simulink model "2DoF Robotic Arm"  (R2024b)
settings: Solver=VariableStepAuto  StartTime=0.0  StopTime=10.0  RelTol=1e-3
model workspace: external: MATLAB File C:\Users\sudhi\Downloads\Sagar_Pathak\IIT_Bhilai\Robotics\Assembly_trial_6_DataFile.m (data not in the file)
undefined symbols (not defined in the file): smiData, X, Y, Z
libraries: sm_lib x19, simulink x7, nesl_utility x3
settings Model: PacingRate=1.100000  Creator=sudhi  LastModifiedBy=sudhi

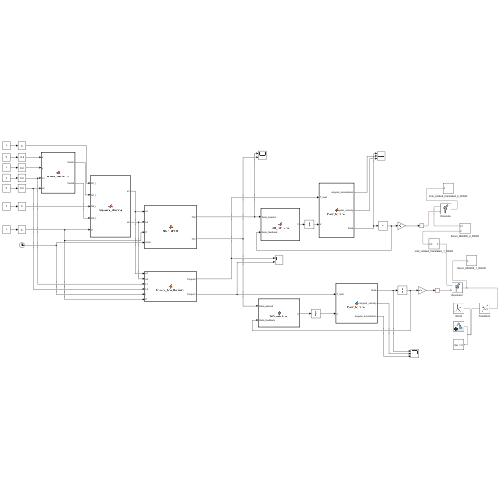
[thumbnail: Simulink's stored preview of the top-level diagram]
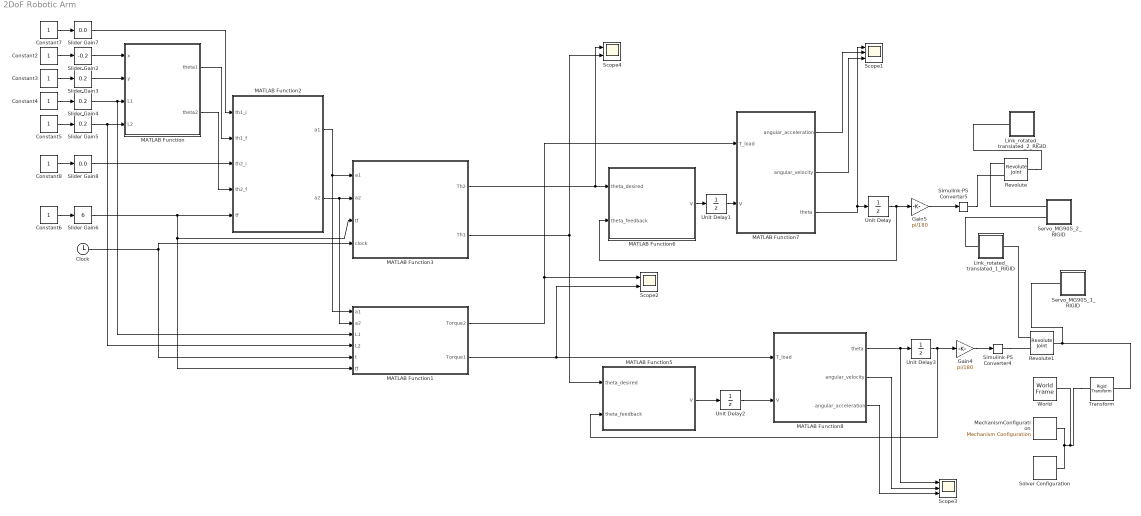
== system 2DoF Robotic Arm ==
  Clock : Clock
  Constant{2..8} (7 alike) : Constant
  Gain4 : Gain  Gain=pi/180
  Gain5 : Gain  Gain=pi/180
  Link_rotated_translated_1_RIGID : Subsystem
  Link_rotated_translated_2_RIGID : Subsystem
  MATLAB Function : MATLAB Function  TreatAsAtomicUnit=on
  MATLAB Function1 : MATLAB Function  TreatAsAtomicUnit=on
  MATLAB Function2 : MATLAB Function  TreatAsAtomicUnit=on
  MATLAB Function3 : MATLAB Function  TreatAsAtomicUnit=on
  MATLAB Function5 : MATLAB Function  TreatAsAtomicUnit=on
  MATLAB Function6 : MATLAB Function  TreatAsAtomicUnit=on
  MATLAB Function7 : MATLAB Function  TreatAsAtomicUnit=on
  MATLAB Function8 : MATLAB Function  TreatAsAtomicUnit=on
  MechanismConfiguration : sm_lib/Utilities/Mechanism Configuration  UniformGravity=Constant  GravityVector=[0 -9.80665 0]  GravityVectorUnits=m/s^2  LinearizationDelta=0.001  JointModeTransitionNonlinearIterations=2
  Revolute : sm_lib/Joints/Revolute Joint  JointMode=Normal  CompositeWrenchDir=FollowerOnBase  CompositeWrenchFrame=BaseFrame  SenseConstraintForce=off  SenseConstraintTorque=off  SenseTotalForce=off  SenseTotalTorque=off  PositionTargetSpecify=on  PositionTargetPriority=Low  PositionTargetValue=smiData.RevoluteJoint(1).Rz.Pos  PositionTargetValueUnits=deg  VelocityTargetSpecify=off  VelocityTargetPriority=High  VelocityTargetValue=0  VelocityTargetValueUnits=deg/s  EquilibriumPosition=0  EquilibriumPositionUnits=deg  SpringStiffness=0  SpringStiffnessUnits=N*m/deg  DampingCoefficient=0  DampingCoefficientUnits=N*m/(deg/s)  LowerLimitSpecify=off  LowerLimitBound=-90  LowerLimitBoundUnits=deg  LowerLimitStiffness=1e4  LowerLimitStiffnessUnits=N*m/deg  LowerLimitDamping=10  LowerLimitDampingUnits=N*m/(deg/s)  LowerLimitTransitionRegionWidth=0.1  LowerLimitTransitionRegionWidthUnits=deg  UpperLimitSpecify=off  UpperLimitBound=90  UpperLimitBoundUnits=deg  UpperLimitStiffness=1e4  UpperLimitStiffnessUnits=N*m/deg  UpperLimitDamping=10  UpperLimitDampingUnits=N*m/(deg/s)  UpperLimitTransitionRegionWidth=0.1  UpperLimitTransitionRegionWidthUnits=deg  TorqueActuationMode=ComputedTorque  MotionActuationMode=InputMotion  SensePosition=off  SenseVelocity=off  SenseAcceleration=off  SenseTorqueForce=off  SenseLowerLimitTorqueForce=off  SenseUpperLimitTorqueForce=off
  Revolute1 : sm_lib/Joints/Revolute Joint  JointMode=Normal  CompositeWrenchDir=FollowerOnBase  CompositeWrenchFrame=BaseFrame  SenseConstraintForce=off  SenseConstraintTorque=off  SenseTotalForce=off  SenseTotalTorque=off  PositionTargetSpecify=on  PositionTargetPriority=Low  PositionTargetValue=smiData.RevoluteJoint(1).Rz.Pos  PositionTargetValueUnits=deg  VelocityTargetSpecify=off  VelocityTargetPriority=High  VelocityTargetValue=0  VelocityTargetValueUnits=deg/s  EquilibriumPosition=0  EquilibriumPositionUnits=deg  SpringStiffness=0  SpringStiffnessUnits=N*m/deg  DampingCoefficient=0  DampingCoefficientUnits=N*m/(deg/s)  LowerLimitSpecify=off  LowerLimitBound=-90  LowerLimitBoundUnits=deg  LowerLimitStiffness=1e4  LowerLimitStiffnessUnits=N*m/deg  LowerLimitDamping=10  LowerLimitDampingUnits=N*m/(deg/s)  LowerLimitTransitionRegionWidth=0.1  LowerLimitTransitionRegionWidthUnits=deg  UpperLimitSpecify=off  UpperLimitBound=90  UpperLimitBoundUnits=deg  UpperLimitStiffness=1e4  UpperLimitStiffnessUnits=N*m/deg  UpperLimitDamping=10  UpperLimitDampingUnits=N*m/(deg/s)  UpperLimitTransitionRegionWidth=0.1  UpperLimitTransitionRegionWidthUnits=deg  TorqueActuationMode=ComputedTorque  MotionActuationMode=InputMotion  SensePosition=off  SenseVelocity=off  SenseAcceleration=off  SenseTorqueForce=off  SenseLowerLimitTorqueForce=off  SenseUpperLimitTorqueForce=off
  Scope1 : Scope  NumInputPorts=3
  Scope2 : Scope  NumInputPorts=2
  Scope3 : Scope  NumInputPorts=3
  Scope4 : Scope  NumInputPorts=2
  Servo_MG90S_1_RIGID : Subsystem
  Servo_MG90S_2_RIGID : Subsystem
  Simulink-PS Converter4 : nesl_utility/Simulink-PS Converter  PhysicalDomain=network_engine_domain  SubClassName=ps_input  LeftPortType=input  RightPortType=output  PseudoPeriodic=off  Frequencies=[]  NoiseDistribution=none  NoiseParameters=[]  Unit=1  AffineConversion=off  FilteringAndDerivatives=zero  SimscapeFilterOrder=1  InputFilterTimeConstant=0.001  UdotUserProvided=0
  Simulink-PS Converter5 : nesl_utility/Simulink-PS Converter  PhysicalDomain=network_engine_domain  SubClassName=ps_input  LeftPortType=input  RightPortType=output  PseudoPeriodic=off  Frequencies=[]  NoiseDistribution=none  NoiseParameters=[]  Unit=1  AffineConversion=off  FilteringAndDerivatives=zero  SimscapeFilterOrder=1  InputFilterTimeConstant=0.001  UdotUserProvided=0
  Slider Gain2 : simulink/Math Operations/Slider Gain  gain=-0.2  low=-100  high=100
  Slider Gain3 : simulink/Math Operations/Slider Gain  gain=0.2  low=-10  high=100
  Slider Gain4 : simulink/Math Operations/Slider Gain  gain=0.2  low=0  high=100
  Slider Gain5 : simulink/Math Operations/Slider Gain  gain=0.2  low=0  high=100
  Slider Gain6 : simulink/Math Operations/Slider Gain  gain=6  low=0  high=100
  Slider Gain7 : simulink/Math Operations/Slider Gain  gain=0.0  low=0  high=100
  Slider Gain8 : simulink/Math Operations/Slider Gain  gain=0.0  low=0  high=100
  Solver Configuration : nesl_utility/Solver Configuration  PhysicalDomain=network_engine_domain  SubClassName=solver  LeftPortType=input  RightPortType=generic  Tones=[]  Harmonics=[]  SimulateNoise=off  Profile=off  UseLocalSampling=off  EnableSwitchedLinearOptims=on  FrequencyDomain=off  UseCCode=off  RelTol=0.001  AbsTol=0.001  MinStep=1e-09  ToWorkspace=off  RevertToSquareIcSolve=off  NumHomotopyIterations=100  PhasorMode=off  PhasorModeNumHarmonics=1  ConsistencySolver=NEWTON_XTOL_AFTER_FTOL  IndexReductionMethod=DerivativeReplacement  DoDC=off  ResidualTolerance=1e-09  ConsistencyTolSource=GLOBAL  ConsistencyAbsTol=0.001  ConsistencyRelTol=0.001  ConsistencyTolFactor=0.001  UseLocalSolver=off  LocalSolverChoice=NE_BACKWARD_EULER_ADVANCER  ResolveIndetEquations=on  FunctionEvalNumThread=1  LocalSolverSampleTime=0.001  DoFixedCost=off  MaxNonlinIter=3  MaxModeIter=2  ComputeImpulses=off  ImpulseIterations=2  LinearAlgebra=auto  LinearAlgebraNumThread=0  EquationFormulation=NE_TIME_EF  DelaysMemoryBudget=1024  AutomaticFiltering=on  FilteringTimeConstant=0.001  PartitionStorageMethod=AS_NEEDED  PartitionMemoryBudget=1024  PartitionMethod=ROBUST  MultibodyUseLocalSolver=off  MultibodyLocalSolverChoice=ODE1  MultibodyLocalSolverSampleTime=0.001
  Transform : sm_lib/Frames and Transforms/Rigid Transform  RotationMethod=ArbitraryAxis  FollAlignAxisA=+X  BaseAlignAxisA=+Y  FollAlignAxisB=+Y  BaseAlignAxisB=+Z  RotationStandardAxis=+Z  RotationAngle=smiData.RigidTransform(2).angle  RotationAngleUnits=rad  RotationArbitraryAxis=smiData.RigidTransform(2).axis  RotationSequenceAxes=FollowerAxes  RotationSequence=XYX  RotationSequenceAngles=[0 0 0]  RotationSequenceAnglesUnits=deg  RotationMatrix=[1 0 0;0 1 0;0 0 1]  Quaternion=[1 0 0 0]  TranslationMethod=Cartesian  TranslationCartesianOffset=smiData.RigidTransform(2).translation  TranslationCartesianOffsetUnits=mm  TranslationStandardAxis=+Z  TranslationStandardOffset=0  TranslationStandardOffsetUnits=m  TranslationROffset=0  TranslationROffsetUnits=m  TranslationThetaOffset=0  TranslationThetaOffsetUnits=deg  TranslationZOffset=0  TranslationZOffsetUnits=m
  Unit Delay : UnitDelay  SampleTime=0.01  HasFrameUpgradeWarning=on
  Unit Delay1 : UnitDelay  SampleTime=0.1  HasFrameUpgradeWarning=on
  Unit Delay2 : UnitDelay  SampleTime=0.1  HasFrameUpgradeWarning=on
  Unit Delay3 : UnitDelay  SampleTime=0.01  HasFrameUpgradeWarning=on
  World : sm_lib/Frames and Transforms/World Frame
  wires:
  Slider Gain2/1 -> MATLAB Function/1(x)
  Constant2/1 -> Slider Gain2/1
  Slider Gain3/1 -> MATLAB Function/2(y)
  Constant3/1 -> Slider Gain3/1
  Slider Gain4/1 -> MATLAB Function1/3(L1), MATLAB Function/3(L1)
  Constant4/1 -> Slider Gain4/1
  Slider Gain5/1 -> MATLAB Function/4(L2), MATLAB Function1/4(L2)
  Constant5/1 -> Slider Gain5/1
  MATLAB Function/1(theta1) -> MATLAB Function2/2(th1_f)
  MATLAB Function/2(theta2) -> MATLAB Function2/4(th2_f)
  Constant6/1 -> Slider Gain6/1
  Slider Gain6/1 -> MATLAB Function2/5(tf), MATLAB Function1/6(tf), MATLAB Function3/3(tf)
  Constant7/1 -> Slider Gain7/1
  Slider Gain7/1 -> MATLAB Function2/1(th1_i)
  Constant8/1 -> Slider Gain8/1
  Slider Gain8/1 -> MATLAB Function2/3(th2_i)
  Clock/1 -> MATLAB Function1/5(t), MATLAB Function3/4(clock)
  MATLAB Function3/2(Th1) -> MATLAB Function5/1(theta_desired), Scope4/2
  MATLAB Function3/1(Th2) -> Scope4/1, MATLAB Function6/1(theta_desired)
  MATLAB Function2/2(a2) -> MATLAB Function1/2(a2), MATLAB Function3/2(a2)
  MATLAB Function2/1(a1) -> MATLAB Function3/1(a1), MATLAB Function1/1(a1)
  MATLAB Function1/2(Torque1) -> MATLAB Function8/1(T_load), Scope2/2
  MATLAB Function1/1(Torque2) -> Scope2/1, MATLAB Function7/1(T_load)
  Gain4/1 -> Simulink-PS Converter4/1
  Gain5/1 -> Simulink-PS Converter5/1
  MATLAB Function7/3(theta) -> Scope1/1, Unit Delay/1
  Unit Delay/1 -> MATLAB Function6/2(theta_feedback), Gain5/1
  MATLAB Function6/1(V) -> Unit Delay1/1
  Unit Delay1/1 -> MATLAB Function7/2(V)
  MATLAB Function5/1(V) -> Unit Delay2/1
  Unit Delay3/1 -> Gain4/1, MATLAB Function5/2(theta_feedback)
  MATLAB Function8/1(theta) -> Unit Delay3/1, Scope3/1
  Unit Delay2/1 -> MATLAB Function8/2(V)
  MATLAB Function7/2(angular_velocity) -> Scope1/3
  MATLAB Function7/1(angular_acceleration) -> Scope1/2
  MATLAB Function8/2(angular_velocity) -> Scope3/2
  MATLAB Function8/3(angular_acceleration) -> Scope3/3
  connections:
  Transform/LConn1 -- MechanismConfiguration/RConn1 -- Solver Configuration/RConn1 -- World/RConn1
  Revolute1/LConn1 -- Link_rotated_translated_1_RIGID/RConn1
  Revolute1/RConn1 -- Transform/RConn1 -- Servo_MG90S_1_RIGID/LConn1
  Link_rotated_translated_1_RIGID/LConn1 -- Servo_MG90S_2_RIGID/LConn2
  Servo_MG90S_2_RIGID/LConn1 -- Revolute/LConn1
  Revolute/RConn1 -- Link_rotated_translated_2_RIGID/LConn1
  Simulink-PS Converter4/RConn1 -- Revolute1/LConn2
  Simulink-PS Converter5/RConn1 -- Revolute/LConn2

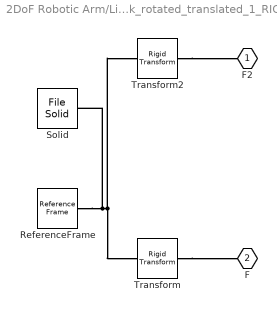
== system 2DoF Robotic Arm/Link_rotated_translated_1_RIGID ==
  ReferenceFrame : sm_lib/Frames and Transforms/Reference Frame
  Solid : sm_lib/Body Elements/File Solid  ExtGeomFileName=Link_rotated_translated_Default_sldprt.STEP  UnitType=FromFile  ExtGeomFileUnits=m  StepReaderType=HEX  ExportConvexHullGeometry=off  InertiaType=Custom  BasedOnType=DensityFromFile  Density=1000  DensityUnits=kg/m^3  Mass=smiData.Solid(1).mass  MassUnits=kg  CenterOfMass=smiData.Solid(1).CoM  CenterOfMassUnits=mm  MomentsOfInertia=smiData.Solid(1).MoI  MomentsOfInertiaUnits=kg*mm^2  ProductsOfInertia=smiData.Solid(1).PoI  ProductsOfInertiaUnits=kg*mm^2  GraphicType=FromGeometry  MarkerShape=Sphere  MarkerSize=10  GraphicVisPropType=SimpleVisualProperties  GraphicDiffuseColor=smiData.Solid(1).color  GraphicOpacity=smiData.Solid(1).opacity  GraphicSpecularColor=[0.5 0.5 0.5 1.0]  GraphicAmbientColor=[0.15 0.15 0.15 1.0]  GraphicEmissiveColor=[0.0 0.0 0.0 1.0]  GraphicShininess=75  DoExposeReferenceFrame=on  SerializedFrames=<Frames/>
  Transform : sm_lib/Frames and Transforms/Rigid Transform  RotationMethod=ArbitraryAxis  FollAlignAxisA=+X  BaseAlignAxisA=+Y  FollAlignAxisB=+Y  BaseAlignAxisB=+Z  RotationStandardAxis=+Z  RotationAngle=smiData.RigidTransform(1).angle  RotationAngleUnits=rad  RotationArbitraryAxis=smiData.RigidTransform(1).axis  RotationSequenceAxes=FollowerAxes  RotationSequence=XYX  RotationSequenceAngles=[0 0 0]  RotationSequenceAnglesUnits=deg  RotationMatrix=[1 0 0;0 1 0;0 0 1]  Quaternion=[1 0 0 0]  TranslationMethod=Cartesian  TranslationCartesianOffset=smiData.RigidTransform(1).translation  TranslationCartesianOffsetUnits=mm  TranslationStandardAxis=+Z  TranslationStandardOffset=0  TranslationStandardOffsetUnits=m  TranslationROffset=0  TranslationROffsetUnits=m  TranslationThetaOffset=0  TranslationThetaOffsetUnits=deg  TranslationZOffset=0  TranslationZOffsetUnits=m
  Transform2 : sm_lib/Frames and Transforms/Rigid Transform  RotationMethod=ArbitraryAxis  FollAlignAxisA=+X  BaseAlignAxisA=+Y  FollAlignAxisB=+Y  BaseAlignAxisB=+Z  RotationStandardAxis=+Z  RotationAngle=smiData.RigidTransform(5).angle  RotationAngleUnits=rad  RotationArbitraryAxis=smiData.RigidTransform(5).axis  RotationSequenceAxes=FollowerAxes  RotationSequence=XYX  RotationSequenceAngles=[0 0 0]  RotationSequenceAnglesUnits=deg  RotationMatrix=[1 0 0;0 1 0;0 0 1]  Quaternion=[1 0 0 0]  TranslationMethod=Cartesian  TranslationCartesianOffset=smiData.RigidTransform(5).translation  TranslationCartesianOffsetUnits=mm  TranslationStandardAxis=+Z  TranslationStandardOffset=0  TranslationStandardOffsetUnits=m  TranslationROffset=0  TranslationROffsetUnits=m  TranslationThetaOffset=0  TranslationThetaOffsetUnits=deg  TranslationZOffset=0  TranslationZOffsetUnits=m
  F2 : PMIOPort  Side=Left
  F : PMIOPort  Port=2  Side=Right
  connections:
  Solid/RConn1 -- ReferenceFrame/RConn1 -- Transform2/LConn1 -- Transform/LConn1
  Transform/RConn1 -- F/RConn1
  Transform2/RConn1 -- F2/RConn1

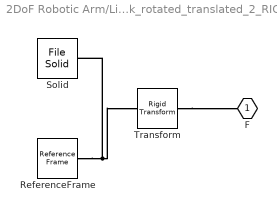
== system 2DoF Robotic Arm/Link_rotated_translated_2_RIGID ==
  ReferenceFrame : sm_lib/Frames and Transforms/Reference Frame
  Solid : sm_lib/Body Elements/File Solid  ExtGeomFileName=Link_rotated_translated_Default_sldprt.STEP  UnitType=FromFile  ExtGeomFileUnits=m  StepReaderType=HEX  ExportConvexHullGeometry=off  InertiaType=Custom  BasedOnType=DensityFromFile  Density=1000  DensityUnits=kg/m^3  Mass=smiData.Solid(1).mass  MassUnits=kg  CenterOfMass=smiData.Solid(1).CoM  CenterOfMassUnits=mm  MomentsOfInertia=smiData.Solid(1).MoI  MomentsOfInertiaUnits=kg*mm^2  ProductsOfInertia=smiData.Solid(1).PoI  ProductsOfInertiaUnits=kg*mm^2  GraphicType=FromGeometry  MarkerShape=Sphere  MarkerSize=10  GraphicVisPropType=SimpleVisualProperties  GraphicDiffuseColor=smiData.Solid(1).color  GraphicOpacity=smiData.Solid(1).opacity  GraphicSpecularColor=[0.5 0.5 0.5 1.0]  GraphicAmbientColor=[0.15 0.15 0.15 1.0]  GraphicEmissiveColor=[0.0 0.0 0.0 1.0]  GraphicShininess=75  DoExposeReferenceFrame=on  SerializedFrames=<Frames/>
  Transform : sm_lib/Frames and Transforms/Rigid Transform  RotationMethod=ArbitraryAxis  FollAlignAxisA=+X  BaseAlignAxisA=+Y  FollAlignAxisB=+Y  BaseAlignAxisB=+Z  RotationStandardAxis=+Z  RotationAngle=smiData.RigidTransform(8).angle  RotationAngleUnits=rad  RotationArbitraryAxis=smiData.RigidTransform(8).axis  RotationSequenceAxes=FollowerAxes  RotationSequence=XYX  RotationSequenceAngles=[0 0 0]  RotationSequenceAnglesUnits=deg  RotationMatrix=[1 0 0;0 1 0;0 0 1]  Quaternion=[1 0 0 0]  TranslationMethod=Cartesian  TranslationCartesianOffset=smiData.RigidTransform(8).translation  TranslationCartesianOffsetUnits=mm  TranslationStandardAxis=+Z  TranslationStandardOffset=0  TranslationStandardOffsetUnits=m  TranslationROffset=0  TranslationROffsetUnits=m  TranslationThetaOffset=0  TranslationThetaOffsetUnits=deg  TranslationZOffset=0  TranslationZOffsetUnits=m
  F : PMIOPort  Side=Left
  connections:
  Solid/RConn1 -- ReferenceFrame/RConn1 -- Transform/LConn1
  Transform/RConn1 -- F/RConn1

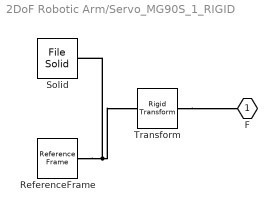
== system 2DoF Robotic Arm/Servo_MG90S_1_RIGID ==
  ReferenceFrame : sm_lib/Frames and Transforms/Reference Frame
  Solid : sm_lib/Body Elements/File Solid  ExtGeomFileName=Servo-MG90S_Default_sldprt.STEP  UnitType=FromFile  ExtGeomFileUnits=m  StepReaderType=HEX  ExportConvexHullGeometry=off  InertiaType=Custom  BasedOnType=DensityFromFile  Density=1000  DensityUnits=kg/m^3  Mass=smiData.Solid(2).mass  MassUnits=kg  CenterOfMass=smiData.Solid(2).CoM  CenterOfMassUnits=mm  MomentsOfInertia=smiData.Solid(2).MoI  MomentsOfInertiaUnits=kg*mm^2  ProductsOfInertia=smiData.Solid(2).PoI  ProductsOfInertiaUnits=kg*mm^2  GraphicType=FromGeometry  MarkerShape=Sphere  MarkerSize=10  GraphicVisPropType=SimpleVisualProperties  GraphicDiffuseColor=smiData.Solid(2).color  GraphicOpacity=smiData.Solid(2).opacity  GraphicSpecularColor=[0.5 0.5 0.5 1.0]  GraphicAmbientColor=[0.15 0.15 0.15 1.0]  GraphicEmissiveColor=[0.0 0.0 0.0 1.0]  GraphicShininess=75  DoExposeReferenceFrame=on  SerializedFrames=<Frames/>
  Transform : sm_lib/Frames and Transforms/Rigid Transform  RotationMethod=ArbitraryAxis  FollAlignAxisA=+X  BaseAlignAxisA=+Y  FollAlignAxisB=+Y  BaseAlignAxisB=+Z  RotationStandardAxis=+Z  RotationAngle=smiData.RigidTransform(3).angle  RotationAngleUnits=rad  RotationArbitraryAxis=smiData.RigidTransform(3).axis  RotationSequenceAxes=FollowerAxes  RotationSequence=XYX  RotationSequenceAngles=[0 0 0]  RotationSequenceAnglesUnits=deg  RotationMatrix=[1 0 0;0 1 0;0 0 1]  Quaternion=[1 0 0 0]  TranslationMethod=Cartesian  TranslationCartesianOffset=smiData.RigidTransform(3).translation  TranslationCartesianOffsetUnits=mm  TranslationStandardAxis=+Z  TranslationStandardOffset=0  TranslationStandardOffsetUnits=m  TranslationROffset=0  TranslationROffsetUnits=m  TranslationThetaOffset=0  TranslationThetaOffsetUnits=deg  TranslationZOffset=0  TranslationZOffsetUnits=m
  F : PMIOPort  Side=Left
  connections:
  Solid/RConn1 -- ReferenceFrame/RConn1 -- Transform/LConn1
  Transform/RConn1 -- F/RConn1

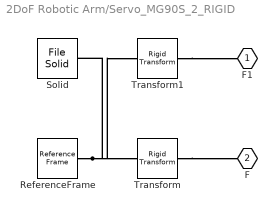
== system 2DoF Robotic Arm/Servo_MG90S_2_RIGID ==
  ReferenceFrame : sm_lib/Frames and Transforms/Reference Frame
  Solid : sm_lib/Body Elements/File Solid  ExtGeomFileName=Servo-MG90S_Default_sldprt.STEP  UnitType=FromFile  ExtGeomFileUnits=m  StepReaderType=HEX  ExportConvexHullGeometry=off  InertiaType=Custom  BasedOnType=DensityFromFile  Density=1000  DensityUnits=kg/m^3  Mass=smiData.Solid(2).mass  MassUnits=kg  CenterOfMass=smiData.Solid(2).CoM  CenterOfMassUnits=mm  MomentsOfInertia=smiData.Solid(2).MoI  MomentsOfInertiaUnits=kg*mm^2  ProductsOfInertia=smiData.Solid(2).PoI  ProductsOfInertiaUnits=kg*mm^2  GraphicType=FromGeometry  MarkerShape=Sphere  MarkerSize=10  GraphicVisPropType=SimpleVisualProperties  GraphicDiffuseColor=smiData.Solid(2).color  GraphicOpacity=smiData.Solid(2).opacity  GraphicSpecularColor=[0.5 0.5 0.5 1.0]  GraphicAmbientColor=[0.15 0.15 0.15 1.0]  GraphicEmissiveColor=[0.0 0.0 0.0 1.0]  GraphicShininess=75  DoExposeReferenceFrame=on  SerializedFrames=<Frames/>
  Transform : sm_lib/Frames and Transforms/Rigid Transform  RotationMethod=ArbitraryAxis  FollAlignAxisA=+X  BaseAlignAxisA=+Y  FollAlignAxisB=+Y  BaseAlignAxisB=+Z  RotationStandardAxis=+Z  RotationAngle=smiData.RigidTransform(6).angle  RotationAngleUnits=rad  RotationArbitraryAxis=smiData.RigidTransform(6).axis  RotationSequenceAxes=FollowerAxes  RotationSequence=XYX  RotationSequenceAngles=[0 0 0]  RotationSequenceAnglesUnits=deg  RotationMatrix=[1 0 0;0 1 0;0 0 1]  Quaternion=[1 0 0 0]  TranslationMethod=Cartesian  TranslationCartesianOffset=smiData.RigidTransform(6).translation  TranslationCartesianOffsetUnits=mm  TranslationStandardAxis=+Z  TranslationStandardOffset=0  TranslationStandardOffsetUnits=m  TranslationROffset=0  TranslationROffsetUnits=m  TranslationThetaOffset=0  TranslationThetaOffsetUnits=deg  TranslationZOffset=0  TranslationZOffsetUnits=m
  Transform1 : sm_lib/Frames and Transforms/Rigid Transform  RotationMethod=ArbitraryAxis  FollAlignAxisA=+X  BaseAlignAxisA=+Y  FollAlignAxisB=+Y  BaseAlignAxisB=+Z  RotationStandardAxis=+Z  RotationAngle=smiData.RigidTransform(7).angle  RotationAngleUnits=rad  RotationArbitraryAxis=smiData.RigidTransform(7).axis  RotationSequenceAxes=FollowerAxes  RotationSequence=XYX  RotationSequenceAngles=[0 0 0]  RotationSequenceAnglesUnits=deg  RotationMatrix=[1 0 0;0 1 0;0 0 1]  Quaternion=[1 0 0 0]  TranslationMethod=Cartesian  TranslationCartesianOffset=smiData.RigidTransform(7).translation  TranslationCartesianOffsetUnits=mm  TranslationStandardAxis=+Z  TranslationStandardOffset=0  TranslationStandardOffsetUnits=m  TranslationROffset=0  TranslationROffsetUnits=m  TranslationThetaOffset=0  TranslationThetaOffsetUnits=deg  TranslationZOffset=0  TranslationZOffsetUnits=m
  F1 : PMIOPort  Side=Left
  F : PMIOPort  Port=2  Side=Left
  connections:
  Solid/RConn1 -- ReferenceFrame/RConn1 -- Transform/LConn1 -- Transform1/LConn1
  Transform/RConn1 -- F/RConn1
  Transform1/RConn1 -- F1/RConn1

== matlab function 2DoF Robotic Arm/MATLAB Function1 ==
  data: Torque2 output; a1 input; Torque1 output; a2 input; L1 input; L2 input; t input; tf input
function [Torque2, Torque1] = Robotic_Arm_Dynamics(a1, a2, L1, L2, t, tf)

    if t < 0
        t = 0;
    elseif t > tf
        t = tf;
    end

    
    g = 9.81;
    m1= 0.1;
    m2= 0.1;
    % Center of mass at L/2
    lc1 = L1 / 2;
    lc2 = L2 / 2;

    % Moments of inertia (rod about center)
    % I1 = (1/12) * m1 * L1^2;
    % I2 = (1/12) * m2 * L2^2;

    % Symbolic expressions for theta, theta_dot, theta_ddot
    th1 = a1(1) + a1(2)*t + a1(3)*t^2 + a1(4)*t^3;
    th2 = a2(1) + a2(2)*t + a2(3)*t^2 + a2(4)*t^3;

    th1dot =  a1(2) + 2*a1(3)*t + 3*a1(4)*t^2;
    th2dot =  a2(2) + 2*a2(3)*t + 3*a2(4)*t^2;

    th1ddot =   2*a1(3) + 2*3*a1(4)*t;
    th2ddot =   2*a2(3) + 2*3*a2(4)*t;

    %% Position of center of mass
    % x1 = lc1 * cos(th1);
    % y1 = lc1 * sin(th1);
    % 
    % x2 = L1 * cos(th1) + lc2 * cos(th1 + th2);
    % y2 = L1 * sin(th1) + lc2 * sin(th1 + th2);

    

    
    
    d_dhoL_dho_th1dot_dt = lc1^2*m1*th1ddot + lc1^2*m2*th1ddot + lc2^2*m2*th1ddot + lc2^2*m2*th2ddot + 2*lc1*lc2*m2*cos(th2)*th1ddot + lc1*lc2*m2*cos(th2)*th2ddot - 2*lc1*lc2*m2*sin(th2)*th1dot*th2dot - lc1*lc2*m2*sin(th2)*th2dot*th2dot;
    d_dhoL_dho_th2dot_dt = lc2^2*m2*th1ddot + lc2^2*m2*th2ddot + lc1*lc2*m2*cos(th2)*th1ddot - lc1*lc2*m2*sin(th2)*th1dot*th2dot;
    
    dhoL_dho_th1 = - g*m2*(lc2*cos(th1 + th2) + lc1*cos(th1)) - lc1*g*m1*cos(th1);
    dhoL_dho_th2 = - (m2*(2*lc2*sin(th1 + th2)*(lc1*th1dot*cos(th1) + lc2*cos(th1 + th2)*(th1dot + th2dot))*(th1dot + th2dot) - 2*lc2*cos(th1 + th2)*(lc1*th1dot*sin(th1) + lc2*sin(th1 + th2)*(th1dot + th2dot))*(th1dot + th2dot)))/2 - lc2*g*m2*cos(th1 + th2);
    
    Torque1 = d_dhoL_dho_th1dot_dt - dhoL_dho_th1
    Torque2 = d_dhoL_dho_th2dot_dt - dhoL_dho_th2

end

== matlab function 2DoF Robotic Arm/MATLAB Function ==
  data: theta1 output; x input; theta2 output; y input; L1 input; L2 input
function [theta1, theta2]= inverse_kinematics(x,y, L1, L2)
% this function takes The final desired coordinates of the RA 
% as inputs and generates required angles to achieve them as output

    r_squared = x^2 + y^2;
    
    % Check reachability
    if sqrt(r_squared) > (L1 + L2) || sqrt(r_squared) < abs(L1 - L2)
        error('Target is out of reach for the given arm dimensions.');
    end
    
    % Compute theta2
    cos_theta2 = (r_squared - L1^2 - L2^2) / (2 * L1 * L2);
    theta2 = acos(cos_theta2);  % Elbow-down solution

    % Compute theta1
    k1 = L1 + L2 * cos(theta2);
    k2 = L2 * sin(theta2);
    theta1 =  (atan2(k2, k1) - atan2(y, x));

    % Optional: return angles in degrees
    theta1 = rad2deg(theta1);
    theta2 = rad2deg(theta2);
    fprintf("Calculated angle %.2f, %.2f",theta1, theta2 );
end

== matlab function 2DoF Robotic Arm/MATLAB Function2 ==
  data: th1_i input; th1_f input; th2_i input; th2_f input; tf input; a1 output; a2 output
function [ a1 , a2] = Trajectory_planning(th1_i, th1_f, th2_i, th2_f, tf)
%     coder.extrinsic('syms', 'solve', 'subs');
% syms t c0 c1 c2 c3 real
% 
%     % Declare symbolic variables
%     t = syms('t');
%     c0 = syms('c0');
%     c1 = syms('c1');
%     c2 = syms('c2');
%     c3 = syms('c3');
% 
%     % Time interval
%     t0 = 0;
%     tf = time_span;
% 
%     % Define cubic polynomial and its derivative
%     theta = c0 + c1*t + c2*t^2 + c3*t^3;
%     thetadot = diff(theta, t);
% 
%     % Initial and final angular velocities
%     omega1_i = 0; omega1_f = 0;
%     omega2_i = 0; omega2_f = 0;
% 
%     %% Joint 1 trajectory equations
%     eqns_1 = [
%         subs(theta, t, t0) == th1_i;
%         subs(thetadot, t, t0) == omega1_i;
%         subs(theta, t, tf) == th1_f;
%         subs(thetadot, t, tf) == omega1_f;
%     ];
% 
%     S1 = solve(eqns_1, [c0, c1, c2, c3]);
% 
%     % Substitute solution into theta for joint 1
%     omega1 = simplify(subs(theta, [c0, c1, c2, c3], [S1.c0, S1.c1, S1.c2, S1.c3]));
% 
%     %% Joint 2 trajectory equations
%     eqns_2 = [
%         subs(theta, t, t0) == th2_i;
%         subs(thetadot, t, t0) == omega2_i;
%         subs(theta, t, tf) == th2_f;
%         subs(thetadot, t, tf) == omega2_f;
%     ];
% 
%     S2 = solve(eqns_2, [c0, c1, c2, c3]);
% 
%     % Substitute solution into theta for joint 2
%     omega2 = simplify(subs(theta, [c0, c1, c2, c3], [S2.c0, S2.c1, S2.c2, S2.c3]));

    % function [theta1, theta2] = Trajectory_planning(th1_i, th1_f, th2_i, th2_f, tf, t)
% Cubic trajectory planner for two joints
% Inputs:
%   th1_i, th1_f: Initial and final angle for joint 1
%   th2_i, th2_f: Initial and final angle for joint 2
%   tf: total trajectory time
%   t: current time

    % Clamp time to [0, tf] for safety
    % if t < 0
    %     t = 0;
    % elseif t > tf
    %     t = tf;
    % end

    % Boundary velocities
    v0 = 0;
    vf = 0;

    % Time matrix
    T = [1 0 0^2 0^3;
         0 1 2*0 3*0^2;
         1 tf tf^2 tf^3;
         0 1 2*tf 3*tf^2];

    % Solve for joint 1 coefficients
    B1 = [th1_i; v0; th1_f; vf];
    a1 = T \ B1;

    % Solve for joint 2 coefficients
    B2 = [th2_i; v0; th2_f; vf];
    a2 = T \ B2;

    % Evaluate theta1 and theta2 at time t
    % theta1 = a1(1) + a1(2)*t + a1(3)*t^2 + a1(4)*t^3;
    % theta2 = a2(1) + a2(2)*t + a2(3)*t^2 + a2(4)*t^3;
end

== matlab function 2DoF Robotic Arm/MATLAB Function3 ==
  data: Th2 output; Th1 output; a1 input; a2 input; tf input; clock input
function [Th2, Th1 ]= return_angle(a1,  a2, tf, clock)
    
    t = clock;
    
    % Clamp time to [0, tf] for safety
    if t < 0
        t = 0;
    elseif t > tf
        t = tf;
    end

    % Evaluate theta1 and theta2 at time t
    Th1 = a1(1) + a1(2)*t + a1(3)*t^2 + a1(4)*t^3;
    Th2= a2(1) + a2(2)*t + a2(3)*t^2 + a2(4)*t^3;

    % Plotting
    % figure;
    % plot(t, Th1, 'r', 'LineWidth', 1.5); % Red line for Theta1
    % hold on;
    % plot(t, Th2, 'b', 'LineWidth', 1.5); % Blue line for Theta2
    % hold off;

    
end

== matlab function 2DoF Robotic Arm/MATLAB Function5 ==
  data: theta_desired input; V output; theta_feedback input
function V = PID_calculator( theta_desired, theta_feedback)
    % Parameters
    Kp = 1.75;
    Ki = 0.0;
    Kd = 10;

    persistent integral_error prev_error
    if isempty(integral_error)
        integral_error = 0;
        prev_error = 0;
    end

    dt = 0.1;  % Same as Simulink step size
    error = theta_desired - theta_feedback;
    integral_error = integral_error + error * dt;
    derivative_error = (error - prev_error) / dt;
    prev_error = error;

    V = Kp*error + Ki*integral_error + Kd*derivative_error;
    % V = 100;
end

== matlab function 2DoF Robotic Arm/MATLAB Function6 ==
  data: theta_desired input; V output; theta_feedback input
function V = PID_calculator( theta_desired, theta_feedback)
    % Parameters
    Kp = 1.75;
    Ki = 0.0;
    Kd = 10;

    persistent integral_error prev_error
    if isempty(integral_error)
        integral_error = 0;
        prev_error = 0;
    end

    dt = 0.1;  % Same as Simulink step size
    error = theta_desired - theta_feedback;
    integral_error = integral_error + error * dt;
    derivative_error = (error - prev_error) / dt;
    prev_error = error;

    V = Kp*error + Ki*integral_error + Kd*derivative_error;
    % V = 100;
end

== matlab function 2DoF Robotic Arm/MATLAB Function7 ==
  data: angular_acceleration output; angular_velocity output; T_load input; V input; theta output
function [angular_acceleration , angular_velocity,theta ]= Motor_Dynamic(T_load, V)

    
    
    % T_load = 0
    % Motor constants
    J = 0.824;
    B = 0.0079;
    K = 1.3908;
    R = 1.7;
    L = 0.0163;

    b = (R * J + B * L);
    c = (R * B + K^2);
    e = (L * J);
    d = T_load * R;

    persistent omega omega_dot theta_val
    if isempty(omega)
        omega = 0;
        omega_dot = 0;
        theta_val = 0;
    end

    dt = 0.01;
    omega_ddot = ((V*K - b * omega_dot - c * omega - d)/e);
    omega_dot = omega_dot + omega_ddot * dt;
    omega = omega + omega_dot * dt;
    theta_val = theta_val + omega * dt;

    theta = theta_val;
    angular_velocity = omega;
    angular_acceleration = omega_dot;

    % x(1) = theta;
    % x(2)= omega;
    % x(3)= omega_dot;
    % 
    % xdot = [x(2);
    %     x(3);
    %     ((V*K - b * x(3) - c * x(2) - d)/e);];
end

== matlab function 2DoF Robotic Arm/MATLAB Function8 ==
  data: T_load input; V input; theta output; angular_velocity output; angular_acceleration output
function [theta, angular_velocity, angular_acceleration] = Motor_Dynamic(T_load, V)
% function [theta,angular_velocity,angular_acceleration] = Motor_Dynamic(T_load, V)
%     % T_load = 0
%     % Motor constants
%     J = 0.824;
%     B = 0.0079;
%     K = 1.3908;
%     R = 1.7;
%     L = 0.0163;
% 
%     b = (R * J + B * L);
%     c = (R * B + K^2);
%     e = (L * J);
%     d = T_load * R;
% 
%     persistent omega omega_dot theta_val
%     if isempty(omega)
%         omega = 0;
%         omega_dot = 0;
%         theta_val = 0;
%     end
% 
%     dt = 0.01;
%     omega_ddot = ((V*K - b * omega_dot - c * omega - d)/e);
%     omega_dot = omega_dot + omega_ddot * dt;
%     omega = omega + omega_dot * dt;
%     theta_val = theta_val + omega * dt;
% 
%     theta = theta_val;
%     angular_velocity = omega;
%     angular_acceleration = omega_dot;
% 
% 
% 
% end


% function [angular_acceleration , angular_velocity,theta ]= Motor_Dynamic(T_load, V)

    
    
    % T_load = 0
    % Motor constants
    J = 0.824;
    B = 0.0079;
    K = 1.3908;
    R = 1.7;
    L = 0.0163;

    b = (R * J + B * L);
    c = (R * B + K^2);
    e = (L * J);
    d = T_load * R;

    persistent omega omega_dot theta_val
    if isempty(omega)
        omega = 0;
        omega_dot = 0;
        theta_val = 0;
    end

    dt = 0.01;
    omega_ddot = ((V*K - b * omega_dot - c * omega - d)/e);
    omega_dot = omega_dot + omega_ddot * dt;
    omega = omega + omega_dot * dt;
    theta_val = theta_val + omega * dt;

    theta = theta_val;
    angular_velocity = omega;
    angular_acceleration = omega_dot;

    % x(1) = theta;
    % x(2)= omega;
    % x(3)= omega_dot;
    % 
    % xdot = [x(2);
    %     x(3);
    %     ((V*K - b * x(3) - c * x(2) - d)/e);];
end
